simulink model "HIL_Testing_SW_amantest"  (Simulink 7.5)
settings: Solver=ode1  StartTime=0.0  StopTime=Inf  FixedStep=0.001  RelTol=1e-3
PostLoadFcn:
  | , if any(exist('dsrtsu_mdlpostloadfcn', 'file') == [2, 3, 6]), try dsrtsu_mdlpostloadfcn('Execute', bdroot); catch fprintf('Error in PostLoadFcn (dsrtsu_mdlpostloadfcn) for model "%s":\n %s\n', bdroot, lasterr); end, end,
undefined symbols (not defined in the file): CeBSER_Cnt_NumTempAxisPts, ChargeCord, ChargeCord_Control, ChargeToSOCCurr, ChrgCurrLim, CrntSens1Fine, CS_SOCSetPt, CyclerMaxChrgPwr, CyclerMaxDschrgPwr, deltaAhr, Drive_1, Drive_10, Drive_11, Drive_12, Drive_13, Drive_14, Drive_15, Drive_16, Drive_17, Drive_18, Drive_19, Drive_2, Drive_20, Drive_21, Drive_22, Drive_23, Drive_24, Drive_25, Drive_26, Drive_27, Drive_28, Drive_29, Drive_3, Drive_30, Drive_31, Drive_32, Drive_33, Drive_34, Drive_35, Drive_36, Drive_37, Drive_38, Drive_39, Drive_4, Drive_40, Drive_41, Drive_42, Drive_43, Drive_44, Drive_45, Drive_46, Drive_47, Drive_48, Drive_49, Drive_5, Drive_50, Drive_51, Drive_6, Drive_7, Drive_8 ... (+50)
libraries: simulink x129, rtican x50, rti2211sailib x5, rti2211serlib x5, rti2202miolib x3
(part 13 of 23)

== system HIL_Testing_SW_amantest/LionsHeart/Input Processing/Time/DetermineStartTimestamp ==
  Timestamp_A : Inport  OutDataType=fixdt(1, 16)  OutScaling=2^0
  Enable : EnablePort
  StartTimestamp : Outport  OutDataType=fixdt(1, 16)  OutScaling=2^0
  wires:
  Timestamp_A/1 -> StartTimestamp/1

== system HIL_Testing_SW_amantest/LionsHeart/Input Processing/Time/DetermineTimeRunning ==
  Timestamp_A : Inport  OutDataType=fixdt(1, 16)  OutScaling=2^0
  StartTimestamp : Inport  Port=2  OutDataType=fixdt(1, 16)  OutScaling=2^0
  Enable : EnablePort
  Add : Sum  Inputs=+-  OutDataType=fixdt(1, 16)  OutScaling=2^-10
  Constant : Constant  Value=1000  OutDataType=fixdt(1, 16)  OutScaling=2^0
  Divide : Product  Inputs=*/  OutDataType=fixdt(1, 16)  OutScaling=2^-10
  TimeRunning : Outport  OutDataType=fixdt(1, 16)  OutScaling=2^0
  wires:
  Timestamp_A/1 -> Add/1
  StartTimestamp/1 -> Add/2
  Divide/1 -> TimeRunning/1
  Add/1 -> Divide/1
  Constant/1 -> Divide/2

== system HIL_Testing_SW_amantest/LionsHeart/Input Processing/Voltage Processing/ChargeTermVoltage ==
  BatteryTemp : Inport  OutDataType=fixdt(1, 16)  OutScaling=2^0
  VoltageTarget : Inport  Port=2  OutDataType=fixdt(1, 16)  OutScaling=2^0
  Add : Sum  OutDataType=sfix(16)  OutScaling=2^-10
  Add1 : Sum  Inputs=+-  OutDataType=sfix(16)  OutScaling=2^-10
  Add3 : Sum  OutDataType=sfix(16)  OutScaling=2^-10
  Add4 : Sum  Inputs=+-  OutDataType=sfix(16)  OutScaling=2^-10
  Compare To Zero : simulink/Logic and Bit Operations/Compare To Zero  SystemSampleTime=-1  relop=~=  LogicOutDataTypeMode=uint8  ZeroCross=off
  Compare To Zero1 : simulink/Logic and Bit Operations/Compare To Zero  SystemSampleTime=-1  relop=~=  LogicOutDataTypeMode=uint8  ZeroCross=off
  ConvCellToPack_Volt1 : Subsystem  Tag=1.0
      mask Type: Subsystem
      mask Display:
      | text(.52,.01,char(get_param(gcb,'Tag') ), 'horizontalAlignment','center','verticalAlignment','bottom' )
      | disp(get_param(gcb,'Name'))
  ConvCellToPack_Volt2 : Subsystem  Tag=1.0
      mask Type: Subsystem
      mask Display:
      | text(.52,.01,char(get_param(gcb,'Tag') ), 'horizontalAlignment','center','verticalAlignment','bottom' )
      | disp(get_param(gcb,'Name'))
  Data Store Read : DataStoreRead  DataStoreName=ManualVoltageTerm_Switch  SampleTime=0
  Data Store Read5 : DataStoreRead  DataStoreName=Voltage_Lid  SampleTime=0
  Data Store Write20 : DataStoreWrite  DataStoreName=VoltageTerm  SampleTime=-1
  Data Store Write31 : DataStoreWrite  DataStoreName=VoltageTerm_MaxCell  SampleTime=-1
  Data Type Conversion1 : DataTypeConversion  OutDataTypeMode=single  OutDataType=fixdt(1, 16)  OutScaling=2^0  OutDataTypeStr=single
  Data Type Conversion4 : DataTypeConversion  OutDataTypeMode=single  OutDataType=fixdt(1, 16)  OutScaling=2^0  OutDataTypeStr=single
  LookupChrgVoltageSetPoint_BSE : Subsystem  Tag=x.x
      mask Type: Subsystem
      mask Display:
      | text(.52,.01,char(get_param(gcb,'Tag') ), 'horizontalAlignment','center','verticalAlignment','bottom' )
      | disp(get_param(gcb,'Name'))
  MaxModVoltageOverShoot : Lookup  InputValues=KnBSER_T_BlendTempAxis  Table=KtBSER_U_MaxModChrgSetPtOffst  OutDataType=fixdt(1, 16)  OutScaling=2^0
  Relational Operator : RelationalOperator  Operator=>  LogicOutDataTypeMode=boolean  LogicDataType=fixdt(0, 8)  OutDataTypeStr=boolean
  SOCOffset : Lookup  InputValues=KnHVEM_T_TempAxis  Table=KtSBER_Pct_PackChrgSetPtOffst  OutDataType=fixdt(1, 16)  OutScaling=2^0
  SOCTerm : DataStoreRead  DataStoreName=SOCTerm  SampleTime=0
  SOCTerm1 : DataStoreRead  DataStoreName=ManualVoltageTerm  SampleTime=0
  Switch : Switch  Criteria=u2 > Threshold  OutDataType=fixdt(1, 16)  OutScaling=2^0  OutDataTypeStr=Inherit: Inherit via back propagation
  Switch1 : Switch  Criteria=u2 > Threshold  OutDataType=fixdt(1, 16)  OutScaling=2^0
  Switch3 : Switch  Criteria=u2 > Threshold  OutDataType=fixdt(1, 16)  OutScaling=2^0
  Switch5 : Switch  Criteria=u2 > Threshold  Threshold=0.5  OutDataType=fixdt(1, 16)  OutScaling=2^0
  VOffset1 : Constant  Value=0  OutDataType=fixdt(1, 16)  OutScaling=2^0  OutDataTypeStr=Inherit: Inherit via back propagation
  VoltageOverShoot : Lookup  InputValues=KnHVEM_T_TempAxis  Table=KtBSER_U_PkChrgVSetPtOvrsht  OutDataType=fixdt(1, 16)  OutScaling=2^0
  wires:
  [BatTemp] -> VoltageOverShoot/1
  VoltageOverShoot/1 -> Add/2
  Add/1 -> Switch/3
  ConvCellToPack_Volt1/1(PackLevel_Volt) -> Add/1
  [BatTemp] -> LookupChrgVoltageSetPoint_BSE/2(T)
  LookupChrgVoltageSetPoint_BSE/1(Output Parameter) -> ConvCellToPack_Volt1/1(CellLevel_Volt), [VoltageSet]
  Switch3/1 -> Data Store Write20/1
  Switch/1 -> Switch3/3
  [VoltTarget] -> Compare To Zero/1
  Compare To Zero/1 -> Switch3/2
  [VoltTarget] -> Data Type Conversion4/1
  Data Type Conversion4/1 -> Switch3/1
  [BatTemp] -> MaxModVoltageOverShoot/1
  MaxModVoltageOverShoot/1 -> Add3/2
  [VoltageSet] -> Add3/1
  Add3/1 -> ConvCellToPack_Volt2/1(CellLevel_Volt)
  Data Store Read5/1 -> Relational Operator/2, Switch5/1
  Relational Operator/1 -> Switch5/2
  Switch5/1 -> Add4/1
  VOffset1/1 -> Add4/2
  ConvCellToPack_Volt2/1(PackLevel_Volt) -> Relational Operator/1, Switch5/3
  BatteryTemp/1 -> [BatTemp]
  VoltageTarget/1 -> [VoltTarget]
  SOCTerm1/1 -> Switch/1
  Data Store Read/1 -> Switch/2
  [VoltTarget] -> Compare To Zero1/1
  Compare To Zero1/1 -> Switch1/2
  [VoltTarget] -> Data Type Conversion1/1
  Data Type Conversion1/1 -> Switch1/1
  Add4/1 -> Switch1/3
  Switch1/1 -> Data Store Write31/1
  SOCTerm/1 -> Add1/1
  SOCOffset/1 -> Add1/2
  Add1/1 -> LookupChrgVoltageSetPoint_BSE/1(SocACChrg)
  [BatTemp] -> SOCOffset/1

== system HIL_Testing_SW_amantest/LionsHeart/Input Processing/Voltage Processing/MaxCell_System ==
  MaxCell : Inport  OutDataType=fixdt(1, 16)  OutScaling=2^0
  NumberOfCells : DataStoreRead  DataStoreName=NumberOfCells  SampleTime=0
  mult1 : Product  Inputs=**  OutDataType=fixdt(1, 16)  OutScaling=2^-10
  PackVolt_MaxCell : Outport  OutDataType=fixdt(1, 16)  OutScaling=2^0
  wires:
  mult1/1 -> PackVolt_MaxCell/1
  MaxCell/1 -> mult1/2
  NumberOfCells/1 -> mult1/1

== system HIL_Testing_SW_amantest/LionsHeart/Input Processing/Voltage Processing/MinCell_System ==
  MinCell : Inport  OutDataType=fixdt(1, 16)  OutScaling=2^0
  NumberOfCells : DataStoreRead  DataStoreName=NumberOfCells  SampleTime=0
  mult1 : Product  Inputs=**  OutDataType=fixdt(1, 16)  OutScaling=2^-10
  PackVolt_MinCell : Outport  OutDataType=fixdt(1, 16)  OutScaling=2^0
  wires:
  NumberOfCells/1 -> mult1/1
  MinCell/1 -> mult1/2
  mult1/1 -> PackVolt_MinCell/1

== system HIL_Testing_SW_amantest/LionsHeart/Input Processing/Voltage Processing/PackVLid ==
  PackVoltage : Inport  OutDataType=fixdt(1, 16)  OutScaling=2^0
  BatteryTemp : Inport  Port=2  OutDataType=fixdt(1, 16)  OutScaling=2^0
  MaxCellPackEquiv : Inport  Port=3  OutDataType=fixdt(1, 16)  OutScaling=2^0
  HVBatVltUpLmt_CAN : Inport  Port=4  OutDataType=fixdt(1, 16)  OutScaling=2^0
  Add1 : Sum  Inputs=+-  OutDataType=fixdt(1, 16)  OutScaling=2^-10  OutDataTypeStr=Inherit: Inherit via back propagation
  Add5 : Sum  Inputs=+-  OutDataType=fixdt(1, 16)  OutScaling=2^-10  OutDataTypeStr=Inherit: Inherit via back propagation
  ConvCellToPack_Volt4 : Subsystem  Tag=1.0
      mask Type: Subsystem
      mask Display:
      | text(.52,.01,char(get_param(gcb,'Tag') ), 'horizontalAlignment','center','verticalAlignment','bottom' )
      | disp(get_param(gcb,'Name'))
  Data Store Read : DataStoreRead  DataStoreName=VlidOffset_Switch  SampleTime=0
  Data Store Read1 : DataStoreRead  DataStoreName=VLim_Switch  SampleTime=0
  Data Store Read2 : DataStoreRead  DataStoreName=VLim_Switch  SampleTime=0
  Data Store Read3 : DataStoreRead  DataStoreName=Static_Cell  SampleTime=0
  Data Store Write30 : DataStoreWrite  DataStoreName=Voltage_Lid_Cell  SampleTime=-1
  Data Store Write32 : DataStoreWrite  DataStoreName=Voltage_Lid  SampleTime=-1
  Switch{1..3,7} (4 alike) : Switch  Threshold=.5  OutDataType=fixdt(1, 16)  OutScaling=2^0  OutDataTypeStr=Inherit: Inherit via back propagation
  VoltageLid : Lookup  InputValues=[-30 -20 -10 0 10 20 30 40 50]  Table=[Voltage_Lid]  OutDataType=fixdt(1, 16)  OutScaling=2^0
  wires:
  VoltageLid/1 -> ConvCellToPack_Volt4/1(CellLevel_Volt)
  Add5/1 -> Switch7/1
  ConvCellToPack_Volt4/1(PackLevel_Volt) -> Add5/1, Switch7/3, Switch1/1, [Static]
  BatteryTemp/1 -> VoltageLid/1
  Data Store Read/1 -> Switch7/2
  PackVoltage/1 -> Add1/1
  MaxCellPackEquiv/1 -> Add1/2
  Add1/1 -> Add5/2
  Data Store Read1/1 -> Switch1/2
  HVBatVltUpLmt_CAN/1 -> [HVBatVltUpLmt_CAN]
  Switch7/1 -> Switch2/1
  Switch2/1 -> Data Store Write32/1
  Data Store Read2/1 -> Switch2/2
  [HVBatVltUpLmt_CAN] -> Switch2/3
  [HVBatVltUpLmt_CAN] -> Switch1/3
  Switch3/1 -> Data Store Write30/1
  [VoltageLid] -> Switch3/3
  [Static] -> Switch3/1
  Data Store Read3/1 -> Switch3/2
  Switch1/1 -> [VoltageLid]

== system HIL_Testing_SW_amantest/LionsHeart/Input Processing/Voltage Processing/PackVfloor ==
  PackVoltage : Inport  OutDataType=fixdt(1, 16)  OutScaling=2^0
  BatteryTemp : Inport  Port=2  OutDataType=fixdt(1, 16)  OutScaling=2^0
  MinSectionVoltage : Inport  Port=3  OutDataType=fixdt(1, 16)  OutScaling=2^0
  MinCellPackEquiv : Inport  Port=4  OutDataType=fixdt(1, 16)  OutScaling=2^0
  HVBatVltLwLmt_CAN : Inport  Port=5  OutDataType=fixdt(1, 16)  OutScaling=2^0
  Add2 : Sum  OutDataType=fixdt(1, 16)  OutScaling=2^-10  OutDataTypeStr=Inherit: Inherit via back propagation
  Compare To Constant : simulink/Logic and Bit Operations/Compare To Constant  SystemSampleTime=-1  relop===  const=3.0  LogicOutDataTypeMode=uint8
  ConvCellToPack_Volt3 : Subsystem  Tag=1.0
      mask Type: Subsystem
      mask Display:
      | text(.52,.01,char(get_param(gcb,'Tag') ), 'horizontalAlignment','center','verticalAlignment','bottom' )
      | disp(get_param(gcb,'Name'))
  Data Store Read1 : DataStoreRead  DataStoreName=VLim_Switch  SampleTime=0
  Data Store Read2 : DataStoreRead  DataStoreName=VfloorOffset_Switch  SampleTime=0
  Data Store Read3 : DataStoreRead  DataStoreName=Static_Cell  SampleTime=0
  Data Store Write29 : DataStoreWrite  DataStoreName=Voltage_Floor_Cell  SampleTime=-1
  Data Store Write3 : DataStoreWrite  DataStoreName=Voltage_Floor  SampleTime=-1
  EREV : Subsystem
  FloorGain : Constant  OutDataType=fixdt(1, 16)  OutScaling=2^0
  Logical Operator : Logic  Operator=NOT  AllPortsSameDT=off  OutDataTypeMode=boolean  LogicDataType=fixdt(0, 8)  OutDataTypeStr=boolean
  Merge : Merge
  Multiplier : Product  Inputs=**  OutDataType=fixdt(1, 16)  OutScaling=2^-10
  Program : DataStoreRead  DataStoreName=Program  SampleTime=0
  Subsystem1 : Subsystem
  Subtract : Sum  Inputs=+-  OutDataType=fixdt(1, 16)  OutScaling=2^-10
  Subtract1 : Sum  Inputs=+-  OutDataType=fixdt(1, 16)  OutScaling=2^-10
  Switch1 : Switch  Threshold=.5  OutDataType=fixdt(1, 16)  OutScaling=2^0  OutDataTypeStr=Inherit: Inherit via back propagation
  Switch2 : Switch  Threshold=.5  OutDataType=fixdt(1, 16)  OutScaling=2^0  OutDataTypeStr=Inherit: Inherit via back propagation
  Switch4 : Switch  Threshold=.5  OutDataType=fixdt(1, 16)  OutScaling=2^0  OutDataTypeStr=Inherit: Inherit via back propagation
  VoltageFloor : Lookup  InputValues=[-30 -20 -10 0 10 20 30 40 50]  Table=[VoltageFloor]  OutDataType=fixdt(1, 16)  OutScaling=2^0
  wires:
  [VoltageFloor] -> Switch4/3, Add2/2
  Add2/1 -> Switch4/1
  Switch4/1 -> Data Store Write3/1
  VoltageFloor/1 -> ConvCellToPack_Volt3/1(CellLevel_Volt)
  BatteryTemp/1 -> VoltageFloor/1
  Data Store Read2/1 -> Switch4/2
  Subtract/1 -> [MinCellOffset]
  MinCellPackEquiv/1 -> Subtract/2
  PackVoltage/1 -> [PackVoltage]
  [PackVoltage] -> Subtract1/1
  [PackVoltage] -> Subtract/1
  MinSectionVoltage/1 -> Subtract1/2
  Subtract1/1 -> [MinSectionOffset]
  Program/1 -> Compare To Constant/1
  [MinCellOffset] -> EREV/1(MinCellOffset)
  [MinSectionOffset] -> EREV/2(MinSectionOffset)
  EREV/1(VoltageFloorOffset_EREV) -> Merge/1
  Merge/1 -> [PackVfloorOffset]
  Compare To Constant/1 -> [Trigger]
  [Trigger] -> EREV/Enable
  Logical Operator/1 -> Subsystem1/Enable
  [Trigger] -> Logical Operator/1
  Subsystem1/1(VoltageFloorOffset) -> Merge/2
  [MinCellOffset] -> Subsystem1/1(MinCellOffset)
  ConvCellToPack_Volt3/1(PackLevel_Volt) -> Switch1/1, [Static]
  Switch1/1 -> [VoltageFloor]
  Data Store Read1/1 -> Switch1/2
  HVBatVltLwLmt_CAN/1 -> Switch1/3
  [PackVfloorOffset] -> Multiplier/2
  Multiplier/1 -> Add2/1
  FloorGain/1 -> Multiplier/1
  Switch2/1 -> Data Store Write29/1
  [VoltageFloor] -> Switch2/3
  [Static] -> Switch2/1
  Data Store Read3/1 -> Switch2/2

== system HIL_Testing_SW_amantest/LionsHeart/Input Processing/Voltage Processing/Voltage Control Select ==
  PackVoltage : Inport  OutDataType=fixdt(1, 16)  OutScaling=2^0
  CyclerVoltage : Inport  Port=2  OutDataType=fixdt(1, 16)  OutScaling=2^0
  SOCTerm1 : DataStoreRead  DataStoreName=UsePackSensor  SampleTime=0
  Switch5 : Switch  Criteria=u2 > Threshold  Threshold=0.5  OutDataType=fixdt(1, 16)  OutScaling=2^0  OutDataTypeStr=Inherit: Inherit via back propagation
  Voltage_Cntrl : Outport  OutDataType=fixdt(1, 16)  OutScaling=2^0
  wires:
  CyclerVoltage/1 -> Switch5/3
  PackVoltage/1 -> Switch5/1
  Switch5/1 -> Voltage_Cntrl/1
  SOCTerm1/1 -> Switch5/2

== system HIL_Testing_SW_amantest/RTI Data/RTI Data Store/RTI Data Store/RTI Data Store ==
  RTI Data Store : Subsystem
      mask Type: RTI_DATA_STORE
      mask Description:
      | RTI Data Store Block. This block is used by RTI to store internal model dependent data. Deleting this block will result in data loss.
      | 
      | NEVER DELETE, COPY, OR MODIFY THIS BLOCK!
      mask Help:
      | RTI Data Store Block. This block is used by RTI to store internal model dependent data. Deleting this block will result in data loss.
      | 
      | NEVER DELETE, COPY, OR MODIFY THIS BLOCK!
      mask Display: text(0.5, 0.5, ' ', 'HorizontalAlignment', 'center');

== system HIL_Testing_SW_amantest/RX/Read BAS3/PID_Reads/BatTempSub ==
  In : Inport  OutDataType=fixdt(1, 16)  OutScaling=2^0
  Enable : EnablePort
  Constant : Constant  Value=40  OutDataType=fixdt(1, 16)  OutScaling=2^0
  Fcn : Fcn  Expr=u(2)
  Subtract : Sum  Inputs=+-  OutDataType=fixdt(1, 16)  OutScaling=2^-10
  BatTemp : Outport  OutDataType=fixdt(1, 16)  OutScaling=2^0
  wires:
  In/1 -> Fcn/1
  Subtract/1 -> BatTemp/1
  Constant/1 -> Subtract/2
  Fcn/1 -> Subtract/1

== system HIL_Testing_SW_amantest/RX/Read BAS3/PID_Reads/MaxCellSub ==
  In : Inport  OutDataType=fixdt(1, 16)  OutScaling=2^0
  Enable : EnablePort
  Fcn : Fcn  Expr=256*u(2)+u(1)
  PIDConvert : Fcn  Expr=u(1)*.0006
  MaxCell : Outport  OutDataType=fixdt(1, 16)  OutScaling=2^0
  wires:
  In/1 -> Fcn/1
  Fcn/1 -> PIDConvert/1
  PIDConvert/1 -> MaxCell/1

== system HIL_Testing_SW_amantest/RX/Read BAS3/PID_Reads/MinCellSub ==
  In : Inport  OutDataType=fixdt(1, 16)  OutScaling=2^0
  Enable : EnablePort
  Fcn : Fcn  Expr=256*u(2)+u(1)
  PIDConvert : Fcn  Expr=u(1)*.0006
  MinCell : Outport  OutDataType=fixdt(1, 16)  OutScaling=2^0
  wires:
  In/1 -> Fcn/1
  Fcn/1 -> PIDConvert/1
  PIDConvert/1 -> MinCell/1

== system HIL_Testing_SW_amantest/RX/Read BAS3/PID_Reads/Subsystem ==
  PID_Index : Inport  OutDataType=fixdt(1, 16)  OutScaling=2^0
  DgnInf_{1..8} (8 alike) : MultiPortSwitch  zeroidx=off  OutDataType=fixdt(1, 16)  OutScaling=2^0
  Transmit1 : Constant  Value=3  OutDataType=fixdt(1, 16)  OutScaling=2^0  OutDataTypeStr=Inherit: Inherit via back propagation
  Transmit10 : Constant  Value=34  OutDataType=fixdt(1, 16)  OutScaling=2^0  OutDataTypeStr=Inherit: Inherit via back propagation
  Transmit11 : Constant  Value=67  OutDataType=fixdt(1, 16)  OutScaling=2^0  OutDataTypeStr=Inherit: Inherit via back propagation
  Transmit12 : Constant  Value=43  OutDataType=fixdt(1, 16)  OutScaling=2^0  OutDataTypeStr=Inherit: Inherit via back propagation
  Transmit{5..8,13..16,21..24} (12 alike) : Constant  Value=00  OutDataType=fixdt(1, 16)  OutScaling=2^0  OutDataTypeStr=Inherit: Inherit via back propagation
  Transmit17 : Constant  Value=3  OutDataType=fixdt(1, 16)  OutScaling=2^0  OutDataTypeStr=Inherit: Inherit via back propagation
  Transmit18 : Constant  Value=34  OutDataType=fixdt(1, 16)  OutScaling=2^0  OutDataTypeStr=Inherit: Inherit via back propagation
  Transmit19 : Constant  Value=67  OutDataType=fixdt(1, 16)  OutScaling=2^0  OutDataTypeStr=Inherit: Inherit via back propagation
  Transmit2 : Constant  Value=34  OutDataType=fixdt(1, 16)  OutScaling=2^0  OutDataTypeStr=Inherit: Inherit via back propagation
  Transmit20 : Constant  Value=79  OutDataType=fixdt(1, 16)  OutScaling=2^0  OutDataTypeStr=Inherit: Inherit via back propagation
  Transmit3 : Constant  Value=67  OutDataType=fixdt(1, 16)  OutScaling=2^0  OutDataTypeStr=Inherit: Inherit via back propagation
  Transmit4 : Constant  Value=41  OutDataType=fixdt(1, 16)  OutScaling=2^0  OutDataTypeStr=Inherit: Inherit via back propagation
  Transmit9 : Constant  Value=3  OutDataType=fixdt(1, 16)  OutScaling=2^0  OutDataTypeStr=Inherit: Inherit via back propagation
  Dgn8 : Outport  OutDataType=fixdt(1, 16)  OutScaling=2^0
  Dgn7 : Outport  Port=2  OutDataType=fixdt(1, 16)  OutScaling=2^0
  Dgn6 : Outport  Port=3  OutDataType=fixdt(1, 16)  OutScaling=2^0
  Dgn5 : Outport  Port=4  OutDataType=fixdt(1, 16)  OutScaling=2^0
  Dgn4 : Outport  Port=5  OutDataType=fixdt(1, 16)  OutScaling=2^0
  Dgn3 : Outport  Port=6  OutDataType=fixdt(1, 16)  OutScaling=2^0
  Dgn2 : Outport  Port=7  OutDataType=fixdt(1, 16)  OutScaling=2^0
  Dgn1 : Outport  Port=8  OutDataType=fixdt(1, 16)  OutScaling=2^0
  wires:
  PID_Index/1 -> [PID_Index]
  [PID_Index] -> DgnInf_8/1
  [PID_Index] -> DgnInf_7/1
  [PID_Index] -> DgnInf_6/1
  Transmit1/1 -> DgnInf_8/2
  Transmit2/1 -> DgnInf_7/2
  Transmit3/1 -> DgnInf_6/2
  DgnInf_8/1 -> Dgn8/1
  DgnInf_7/1 -> Dgn7/1
  DgnInf_6/1 -> Dgn6/1
  [PID_Index] -> DgnInf_5/1
  Transmit4/1 -> DgnInf_5/2
  DgnInf_5/1 -> Dgn5/1
  [PID_Index] -> DgnInf_4/1
  Transmit5/1 -> DgnInf_4/2
  DgnInf_4/1 -> Dgn4/1
  [PID_Index] -> DgnInf_3/1
  Transmit6/1 -> DgnInf_3/2
  DgnInf_3/1 -> Dgn3/1
  [PID_Index] -> DgnInf_2/1
  Transmit7/1 -> DgnInf_2/2
  DgnInf_2/1 -> Dgn2/1
  [PID_Index] -> DgnInf_1/1
  Transmit8/1 -> DgnInf_1/2
  DgnInf_1/1 -> Dgn1/1
  Transmit9/1 -> DgnInf_8/3
  Transmit10/1 -> DgnInf_7/3
  Transmit11/1 -> DgnInf_6/3
  Transmit12/1 -> DgnInf_5/3
  Transmit13/1 -> DgnInf_4/3
  Transmit14/1 -> DgnInf_3/3
  Transmit15/1 -> DgnInf_2/3
  Transmit16/1 -> DgnInf_1/3
  Transmit19/1 -> DgnInf_6/4
  Transmit18/1 -> DgnInf_7/4
  Transmit17/1 -> DgnInf_8/4
  Transmit20/1 -> DgnInf_5/4
  Transmit21/1 -> DgnInf_4/4
  Transmit22/1 -> DgnInf_3/4
  Transmit23/1 -> DgnInf_2/4
  Transmit24/1 -> DgnInf_1/4

== system HIL_Testing_SW_amantest/RX/Read EREV/Read HVEM/Current ==
  SensTwo : Inport  OutDataType=sfix(16)  OutScaling=2^0
  SensOne : Inport  Port=2  OutDataType=sfix(16)  OutScaling=2^0
  Data Store Read : DataStoreRead  DataStoreName=CrntSens1Fine  SampleTime=0
  Data Store Read1 : DataStoreRead  DataStoreName=CrntSens1Fine  SampleTime=0
  Enabled Subsystem : Subsystem  TreatAsAtomicUnit=on
  Enabled Subsystem1 : Subsystem  TreatAsAtomicUnit=on
  Logical Operator1 : Logic  Operator=NOT  AllPortsSameDT=off  OutDataTypeMode=boolean  LogicDataType=fixdt(0, 8)  OutDataTypeStr=boolean
  Merge : Merge
  Out1 : Outport  OutDataType=sfix(16)  OutScaling=2^0
  wires:
  Data Store Read/1 -> Enabled Subsystem/Enable
  Data Store Read1/1 -> Logical Operator1/1
  Enabled Subsystem/1(Out1) -> Merge/1
  Enabled Subsystem1/1(Out1) -> Merge/2
  Merge/1 -> Out1/1
  SensTwo/1 -> [SensTwo]
  SensOne/1 -> [SensOne]
  [SensTwo] -> Enabled Subsystem/1(SensTwo)
  [SensTwo] -> Enabled Subsystem1/1(SensTwo)
  [SensOne] -> Enabled Subsystem/2(SensOne)
  [SensOne] -> Enabled Subsystem1/2(SensOne)
  Logical Operator1/1 -> Enabled Subsystem1/Enable

== system HIL_Testing_SW_amantest/RX/Read EREV/Read HVEM/Enabled Subsystem ==
  In1 : Inport  OutDataType=sfix(16)  OutScaling=2^0
  In2 : Inport  Port=2  OutDataType=sfix(16)  OutScaling=2^0
  In3 : Inport  Port=3  OutDataType=sfix(16)  OutScaling=2^0
  In4 : Inport  Port=4  OutDataType=sfix(16)  OutScaling=2^0
  In5 : Inport  Port=5  OutDataType=sfix(16)  OutScaling=2^0
  In6 : Inport  Port=6  OutDataType=sfix(16)  OutScaling=2^0
  Enable : EnablePort
  Add : Sum  Inputs=++++++  OutDataType=sfix(16)  OutScaling=2^-10
  BatTemp : Product  Inputs=*/  OutDataType=sfix(16)  OutScaling=2^-10
  Constant : Constant  Value=6  OutDataType=sfix(16)  OutScaling=2^0
  TempAvg : Outport  OutDataType=sfix(16)  OutScaling=2^0
  wires:
  In1/1 -> Add/1
  In2/1 -> Add/2
  In3/1 -> Add/3
  In4/1 -> Add/4
  In5/1 -> Add/5
  In6/1 -> Add/6
  Add/1 -> BatTemp/1
  Constant/1 -> BatTemp/2
  BatTemp/1 -> TempAvg/1
